simulink model "R7014E_QuadTankSim_LQG"  (R2025b)
settings: Solver=ode4  StartTime=0.0  StopTime=4000  FixedStep=0.01  RelTol=1e-3  EnableMultiTasking=on
values from neighbouring files (symbols this model uses):
  A1 = 28    [matlab_workspace.mat]
  a1 = 0.071    [matlab_workspace.mat]
  A2 = 32    [matlab_workspace.mat]
  a2 = 0.057    [matlab_workspace.mat]
  A3 = 28    [matlab_workspace.mat]
  a3 = 0.071    [matlab_workspace.mat]
  A4 = 32    [matlab_workspace.mat]
  a4 = 0.057    [matlab_workspace.mat]
  g = 981    [matlab_workspace.mat]
  gamma1 = 0.7    [matlab_workspace.mat]
  gamma1_M = 0.7    [matlab_workspace.mat]
  gamma2 = 0.6    [matlab_workspace.mat]
  gamma2_M = 0.6    [matlab_workspace.mat]
  h10_M = 12.3    [matlab_workspace.mat]
  h1_init = 12.3    [matlab_workspace.mat]
  h20_M = 12.8    [matlab_workspace.mat]
  h2_init = 12.8    [matlab_workspace.mat]
  h30_M = 1.6    [matlab_workspace.mat]
  h3_init = 1.6    [matlab_workspace.mat]
  h40_M = 1.4    [matlab_workspace.mat]
  h4_init = 1.4    [matlab_workspace.mat]
  k1 = 3.33    [matlab_workspace.mat]
  k1_M = 3.33    [matlab_workspace.mat]
  k2 = 3.35    [matlab_workspace.mat]
  k2_M = 3.35    [matlab_workspace.mat]
  L = [0.0253903063157  0.00669872251938  -0.00763717131985  17.1775356153; 0.0105780800885  0.0181633124943  21.4339038197  -0.0255525830892]    [matlab_workspace.mat]
  Lr = [4.62710191082  -2.40905188483; -3.22197937318  5.94561996641]    [matlab_workspace.mat]
  Q = gram(G_Pm,'o')    [Gramians_test.m]    (also in matlab_workspace.mat = [1e-08  0  0; 0  1e-08  0; 0  0  10])
  R = 0.1    [matlab_workspace.mat]
  Ts = 0.02    [matlab_workspace.mat]
  u_10_M = 3    [matlab_workspace.mat]
  u_20_M = 3    [matlab_workspace.mat]
undefined symbols (not defined in the file or in its folder): sigbuilder_block
Description:
  | Double tank process simulation model
  | V1.0
  | 
  | Author: Wolfgang Birk, LTU
settings Model: MinMaxOverflowLogging=ForceOff  Creator=wolfgang  LastModifiedBy=kaspe
settings SolverCC: AlgebraicLoopSolver=TrustRegion
settings DataIOCC: LimitDataPoints=on  SaveFormat=Array  SignalLoggingSaveFormat=ModelDataLogs  ReturnWorkspaceOutputs=off
settings OptimizationCC: ExpressionDepthLimit=2147483647.0  LifeSpan=inf
settings DebuggingCC: UnderspecifiedInitializationDetection=Classic  MergeDetectMultiDrivingBlocksExec=none  SolverPrmCheckMsg=warning  FcnCallInpInsideContextMsg=warning  UnconnectedInputMsg=warning  UnconnectedOutputMsg=warning  UnconnectedLineMsg=warning  StateNameClashWarn=warning  SFUnexpectedBacktrackingDiag=warning  SFNoUnconditionalDefaultTransitionDiag=warning  SFExecutionAtInitializationDiag=none  ArithmeticOperatorsInVariantConditions=warning
settings HardwareCC: ProdBitPerPointer=32.0  ProdBitPerSizeT=32.0  ProdBitPerPtrDiffT=32.0  ProdLargestAtomicFloat=None  ProdIntDivRoundTo=Undefined  ProdEndianess=Unspecified  ProdWordSize=32.0  ProdHWDeviceType=32-bit Generic
settings ModelReferenceCC: EnableRefExpFcnMdlSchedulingChecks=on  PropagateSignalLabelsOutOfModel=off
settings SFSimCC: SimUseLocalCustomCode=off  CustomCodeUndefinedFunction=UseInterfaceOnly
settings RTWCC: RTWUseLocalCustomCode=off  GPUComputeCapability=3.5
settings CodeAppCC: StateflowObjectComments=on
settings GRTTargetCC: TargetLangStandard=C89/C90 (ANSI)
settings ConfigComp: CovMetricSettings=dw  CovSaveCumulativeToWorkspaceVar=on  CovSaveSingleToWorkspaceVar=on  CovExternalEMLEnable=off

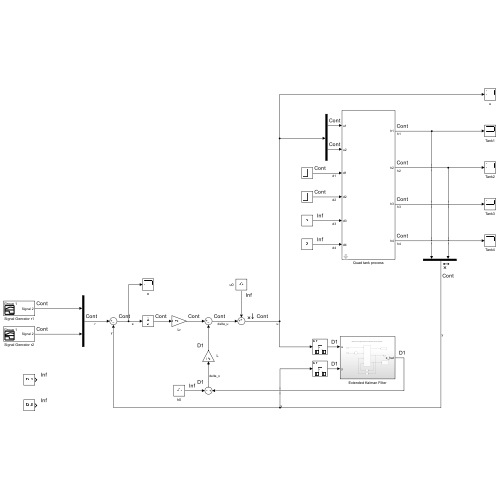
[thumbnail: Simulink's stored preview of the top-level diagram]
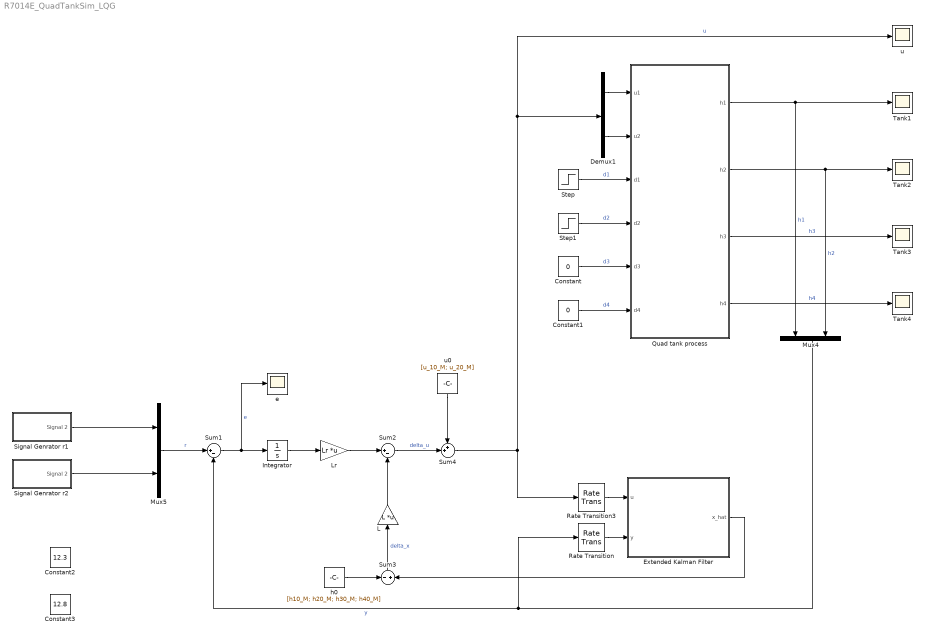
== system R7014E_QuadTankSim_LQG ==
  Constant : Constant  Value=0
  Constant1 : Constant  Value=0
  Constant2 : Constant  Value=12.3
  Constant3 : Constant  Value=12.8
  Demux1 : Demux  Outputs=2
  Extended Kalman Filter : Subsystem
      settings: PortSchema="{\"entries\":[{\"content\":{\"sides\":[{\"content\":{\"connectorIds\":[\"Out1\"]},\"type\":\"ConnectorPlacement.EquallySpacedRectSide\",\"uuid\":\"65fe89cb-b391-4b62-a3a2-a3476ef8bc40\"},{\"content\":{\"connectorIds\":[\"In1\",\"In2\"],\"side\":\"RIGHT\"},\"type\":\"ConnectorPlacement.EquallySpacedRectSide\",\"uuid\":\"bbc6305a-5625-4988-a68f-cd512a800022\"},{\"content\":{\"side\":\"TOP\"},\"type\":\"ConnectorPlacement.EquallySpacedRectSide\",\"uuid\":\"302c5684-92d4-4b6e-95b2-967c1f4e7e8f\"},{\"content\":{\"side\":\"BOTTOM\"},\"type\":\"ConnectorPlacement.EquallySpacedRectSide\",\"uuid\":\"8db0117f-7782-4a07-8d3a-766a48ad4692\"}]},\"type\":\"ConnectorPlacement.EquallySpacedConnector\",\"uuid\":\"a95b63f5-df7a-433e-a941-cc1845937f8d\"}],\"packageUris\":[\"http://schema.mathworks.com/mf0/Connector/R2020b\"],\"version\":\"1.0\"}"
  Integrator : Integrator
  L : Gain  Gain=L  Multiplication=Matrix(K*u)
  Lr : Gain  Gain=Lr  Multiplication=Matrix(K*u)
  Mux4 : Mux  Inputs=2
  Mux5 : Mux  Inputs=2
  Quad tank process : Subsystem  mask{hmax=20, A1=A1, ao1=a1, h10=h1_init, A2=A2, ao2=a2, h20=h2_init, A3=A3, ao3=a3, h30=h3_init, A4=A4, ao4=a4, h40=h4_init, k1=k1_M, k2=k2_M, gamma1=gamma1_M, gamma2=gamma2_M}
      mask prompts: hmax "Tank height (cm)"; A1 "Tank area (cm^2)"; ao1 "Opening area (cm^2)"; h10 "Initial level (cm)"; A2 "Tank area (cm^2)"; ao2 "Opening area (cm^2)"; h20 "Initial level (cm)"; A3 "Tank area (cm^2)"; ao3 "Opening area (cm^2)"; h30 "Initial level (cm)"; A4 "Tank area (cm^2)"; ao4 "Opening area (cm^2)"; h40 "Initial level (cm)"; k1 "Pump1 gain (cm^3/V/s)"; k2 "Pump2 gain (cm^3/V/s)"; gamma1 "Split valve gamma 1"; gamma2 "Split valve gamma 2"
      mask help: Double tank process parameters
      mask DialogControl Container3 Prompt: General parameters
      mask DialogControl ParameterGroupVar Prompt: Tank 1
      mask DialogControl ParameterGroupVar_copy_copy_copy Prompt: Tank 2
      mask DialogControl ParameterGroupVar_copy_copy Prompt: Tank 3
      mask DialogControl ParameterGroupVar_copy Prompt: Tank 4
      mask DialogControl Container4 Prompt: Pump parameters
  Rate Transition : RateTransition  InitialCondition=h1_init  OutPortSampleTime=Ts
  Rate Transition3 : RateTransition  InitialCondition=h2_init  OutPortSampleTime=Ts
  Signal Genrator r1 : Subsystem  Tag=STV Subsys  LoadFcn=sigbuilder_block('load');  StartFcn=sigbuilder_block('start');  StopFcn=sigbuilder_block('stop');  ClipboardFcn=sigbuilder_block('clipboard');  mask(Sigbuilder block){tuvar=[0:10]}
      mask help: Simulink:masks:SigbuilderBlock_MD
      mask init:
      | if ~strcmp(get_param(bdroot(gcbh),'SimulationStatus'),'stopped') tuvar = sigbuilder_block('maskInit'); end
      settings: CopyFcn=sigbuilder_block('copy');  DeleteFcn=sigbuilder_block('delete');  ModelCloseFcn=sigbuilder_block('modelClose');  PreSaveFcn=sigbuilder_block('preSave');  PauseFcn=sigbuilder_block('pause');  ContinueFcn=sigbuilder_block('continue');  NameChangeFcn=sigbuilder_block('namechange');  OpenFcn=sigbuilder_block('open',[289.5 231.75 954.75 575.25 ]);  CloseFcn=sigbuilder_block('close');
      mask Display: plot(0, 0, 100, 100,[2, 2, 32, 32, 2], [68, 8, 8, 68, 68],[32, 2], [38, 38], [32, 19, 2],[53, 60, 44], [32, 17, 17, 2],[16, 16, 31, 31]);txt = getActiveGroup(gcbh);text(2, 100, txt,'verticalAlignment', 'top');
  Signal Genrator r2 : Subsystem  Tag=STV Subsys  LoadFcn=sigbuilder_block('load');  StartFcn=sigbuilder_block('start');  StopFcn=sigbuilder_block('stop');  ClipboardFcn=sigbuilder_block('clipboard');  mask(Sigbuilder block){tuvar=[0:10]}
      mask help: Simulink:masks:SigbuilderBlock_MD
      mask init:
      | if ~strcmp(get_param(bdroot(gcbh),'SimulationStatus'),'stopped') tuvar = sigbuilder_block('maskInit'); end
      settings: CopyFcn=sigbuilder_block('copy');  DeleteFcn=sigbuilder_block('delete');  ModelCloseFcn=sigbuilder_block('modelClose');  PreSaveFcn=sigbuilder_block('preSave');  PauseFcn=sigbuilder_block('pause');  ContinueFcn=sigbuilder_block('continue');  NameChangeFcn=sigbuilder_block('namechange');  OpenFcn=sigbuilder_block('open',[289.5 231.75 954.75 575.25 ]);  CloseFcn=sigbuilder_block('close');
      mask Display: plot(0, 0, 100, 100,[2, 2, 32, 32, 2], [68, 8, 8, 68, 68],[32, 2], [38, 38], [32, 19, 2],[53, 60, 44], [32, 17, 17, 2],[16, 16, 31, 31]);txt = getActiveGroup(gcbh);text(2, 100, txt,'verticalAlignment', 'top');
  Step : Step  Time=1500  After=0.25  SampleTime=0
  Step1 : Step  Time=2700  After=0.25  SampleTime=0
  Sum1 : Sum  Inputs=|+-
  Sum2 : Sum  Inputs=|+-
  Sum3 : Sum  Inputs=-|+
  Sum4 : Sum  Inputs=++|
  Tank{1..4} (4 alike) : Scope
      Tank1 settings: TimeSpan=100  ActiveDisplayYMinimum=11.966385472015087  ActiveDisplayYMaximum=15.227429854493407
      Tank2 settings: TimeSpan=100  ActiveDisplayYMinimum=12.672164495001056  ActiveDisplayYMaximum=12.860911646500954  DataLoggingVariableName=ScopeData3
      Tank3 settings: TimeSpan=100  ActiveDisplayYMinimum=1.57505  ActiveDisplayYMaximum=1.66866
      Tank4 settings: TimeSpan=100  ActiveDisplayYMinimum=1.35987  ActiveDisplayYMaximum=1.45363  DataLoggingVariableName=ScopeData2
  e : Scope
      settings: TimeSpan=100  ActiveDisplayYMinimum=-0.93911904446836725  ActiveDisplayYMaximum=2.3265690426724981  DataLoggingVariableName=ScopeData8
  h0 : Constant  Value=[h10_M; h20_M; h30_M; h40_M]
  u : Scope
      settings: TimeSpan=100  ActiveDisplayYMinimum=-0.83563082318699256  ActiveDisplayYMaximum=10.21135105627962  DataLoggingVariableName=ScopeData4
  u0 : Constant  Value=[u_10_M; u_20_M]
  wires:
  Quad tank process/3(h3) -> Tank3/1  "h3"
  Quad tank process/1(h1) -> Tank1/1, Mux4/1  "h1"
  Step/1 -> Quad tank process/3(d1)  "d1"
  Step1/1 -> Quad tank process/4(d2)  "d2"
  Constant/1 -> Quad tank process/5(d3)  "d3"
  Constant1/1 -> Quad tank process/6(d4)  "d4"
  Quad tank process/2(h2) -> Tank2/1, Mux4/2  "h2"
  Quad tank process/4(h4) -> Tank4/1  "h4"
  Rate Transition/1 -> Extended Kalman Filter/1(y)
  Rate Transition3/1 -> Extended Kalman Filter/2(u)
  Extended Kalman Filter/1(x_hat) -> Sum3/2
  Mux4/1 -> Sum1/2, Rate Transition/1  "y"
  Demux1/1 -> Quad tank process/1(u1)
  Demux1/2 -> Quad tank process/2(u2)
  Mux5/1 -> Sum1/1  "r"
  L/1 -> Sum2/2
  Sum1/1 -> Integrator/1, e/1  "e"
  Sum3/1 -> L/1  "delta_x"
  h0/1 -> Sum3/1
  Sum2/1 -> Sum4/2  "delta_u"
  u0/1 -> Sum4/1
  Sum4/1 -> Rate Transition3/1, Demux1/1, u/1  "u"
  Signal Genrator r1/1(Signal 2) -> Mux5/1
  Signal Genrator r2/1(Signal 2) -> Mux5/2
  Lr/1 -> Sum2/1
  Integrator/1 -> Lr/1

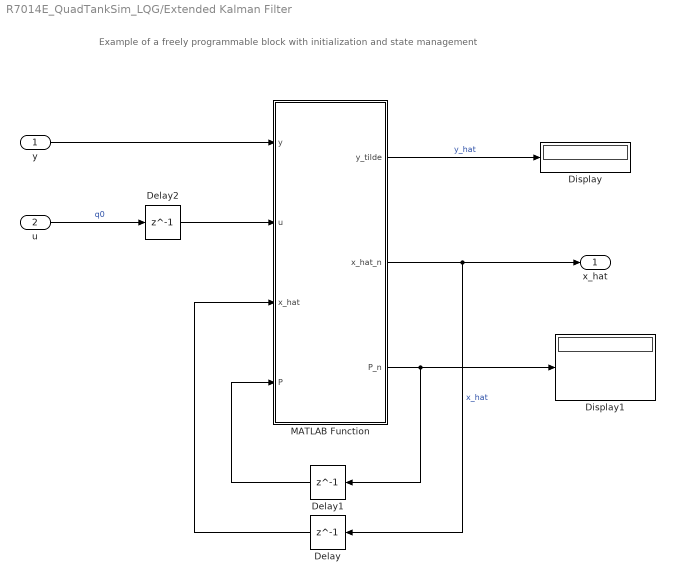
== system R7014E_QuadTankSim_LQG/Extended Kalman Filter ==
  note: Example of a freely programmable block with initialization and state management
  y : Inport
  u : Inport  Port=2
  Delay : Delay  DelayLength=1  InitialCondition=[h1_init, h2_init, h3_init, h4_init]
  Delay1 : Delay  DelayLength=1  InitialCondition=zeros(4)
  Delay2 : Delay  DelayLength=1  InitialCondition=0
  Display : Display
  Display1 : Display
  MATLAB Function : MATLAB Function  TreatAsAtomicUnit=on
  x_hat : Outport
  wires:
  Delay/1 -> MATLAB Function/3(x_hat)
  MATLAB Function/1(y_tilde) -> Display/1  "y_hat"
  MATLAB Function/3(P_n) -> Display1/1, Delay1/1
  Delay1/1 -> MATLAB Function/4(P)
  u/1 -> Delay2/1  "q0"
  MATLAB Function/2(x_hat_n) -> Delay/1, x_hat/1  "x_hat"
  Delay2/1 -> MATLAB Function/2(u)
  y/1 -> MATLAB Function/1(y)

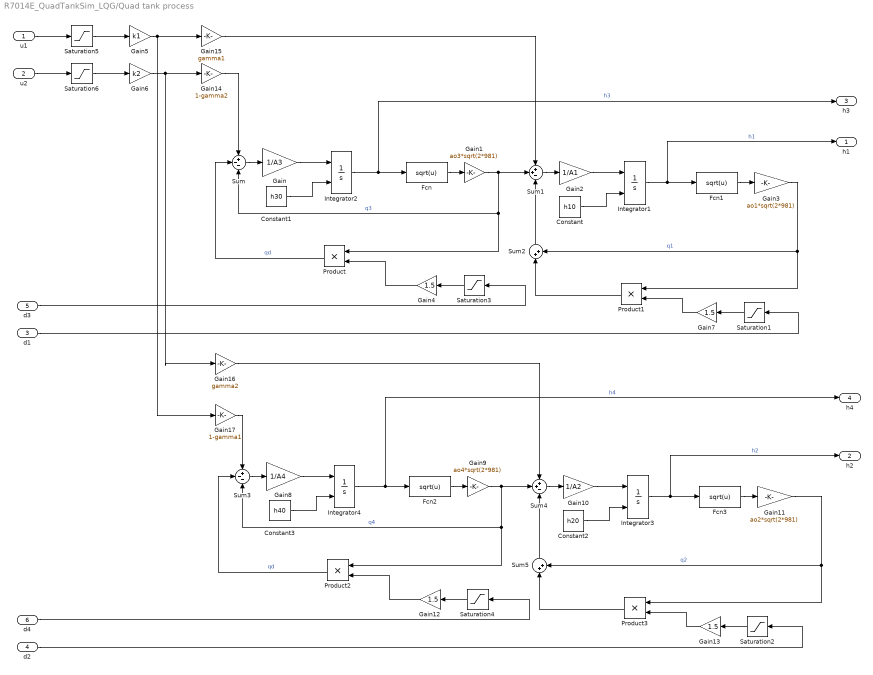
== system R7014E_QuadTankSim_LQG/Quad tank process ==
  u1 : Inport
  u2 : Inport  Port=2
  d1 : Inport  Port=3
  d2 : Inport  Port=4
  d3 : Inport  Port=5
  d4 : Inport  Port=6
  Constant : Constant  Value=h10
  Constant1 : Constant  Value=h30
  Constant2 : Constant  Value=h20
  Constant3 : Constant  Value=h40
  Fcn{,1..3} (4 alike) : Fcn  Expr=sqrt(u)
  Gain : Gain  Gain=1/A3
  Gain1 : Gain  Gain=ao3*sqrt(2*981)
  Gain10 : Gain  Gain=1/A2
  Gain11 : Gain  Gain=ao2*sqrt(2*981)
  Gain{4,7,12..13} (4 alike) : Gain  Gain=1.5
  Gain14 : Gain  Gain=1-gamma2
  Gain15 : Gain  Gain=gamma1
  Gain16 : Gain  Gain=gamma2
  Gain17 : Gain  Gain=1-gamma1
  Gain2 : Gain  Gain=1/A1
  Gain3 : Gain  Gain=ao1*sqrt(2*981)
  Gain5 : Gain  Gain=k1
  Gain6 : Gain  Gain=k2
  Gain8 : Gain  Gain=1/A4
  Gain9 : Gain  Gain=ao4*sqrt(2*981)
  Integrator{1..4} (4 alike) : Integrator  InitialConditionSource=external  LimitOutput=on  UpperSaturationLimit=hmax  LowerSaturationLimit=0
  Product{,1..3} (4 alike) : Product  RndMeth=Zero
  Saturation{1..4} (4 alike) : Saturate  UpperLimit=1  LowerLimit=0
  Saturation5 : Saturate  UpperLimit=10  LowerLimit=0
  Saturation6 : Saturate  UpperLimit=10  LowerLimit=0
  Sum : Sum  Inputs=+--
  Sum1 : Sum  Inputs=++-
  Sum2 : Sum  Inputs=|++
  Sum3 : Sum  Inputs=+--
  Sum4 : Sum  Inputs=++-
  Sum5 : Sum  Inputs=|++
  h1 : Outport  VectorParamsAs1DForOutWhenUnconnected=off
  h2 : Outport  Port=2  VectorParamsAs1DForOutWhenUnconnected=off
  h3 : Outport  Port=3  VectorParamsAs1DForOutWhenUnconnected=off
  h4 : Outport  Port=4  VectorParamsAs1DForOutWhenUnconnected=off
  wires:
  Sum/1 -> Gain/1
  Gain/1 -> Integrator2/1
  Fcn/1 -> Gain1/1
  Gain1/1 -> Product/1, Sum/3, Sum1/2  "q3"
  Sum1/1 -> Gain2/1
  Gain2/1 -> Integrator1/1
  Fcn1/1 -> Gain3/1
  Integrator2/1 -> h3/1, Fcn/1  "h3"
  Product/1 -> Sum/2  "qd"
  d3/1 -> Saturation3/1
  Integrator1/1 -> h1/1, Fcn1/1  "h1"
  Saturation3/1 -> Gain4/1
  Gain4/1 -> Product/2
  u1/1 -> Saturation5/1
  Constant/1 -> Integrator1/2
  Constant1/1 -> Integrator2/2
  u2/1 -> Saturation6/1
  Gain5/1 -> Gain17/1, Gain15/1
  Sum2/1 -> Sum1/3
  Gain3/1 -> Product1/1, Sum2/2  "q1"
  Gain7/1 -> Product1/2
  Saturation1/1 -> Gain7/1
  d1/1 -> Saturation1/1
  Product1/1 -> Sum2/1
  Product3/1 -> Sum5/1
  d2/1 -> Saturation2/1
  Saturation2/1 -> Gain13/1
  Gain13/1 -> Product3/2
  Gain11/1 -> Sum5/2, Product3/1  "q2"
  Sum5/1 -> Sum4/3
  Constant3/1 -> Integrator4/2
  Constant2/1 -> Integrator3/2
  Gain12/1 -> Product2/2
  Saturation4/1 -> Gain12/1
  Integrator3/1 -> Fcn3/1, h2/1  "h2"
  d4/1 -> Saturation4/1
  Product2/1 -> Sum3/2  "qd"
  Integrator4/1 -> h4/1, Fcn2/1  "h4"
  Fcn3/1 -> Gain11/1
  Gain10/1 -> Integrator3/1
  Sum4/1 -> Gain10/1
  Gain9/1 -> Sum4/2, Sum3/3, Product2/1  "q4"
  Fcn2/1 -> Gain9/1
  Gain8/1 -> Integrator4/1
  Sum3/1 -> Gain8/1
  Gain14/1 -> Sum/1
  Gain15/1 -> Sum1/1
  Gain6/1 -> Gain16/1, Gain14/1
  Gain16/1 -> Sum4/1
  Gain17/1 -> Sum3/1
  Saturation5/1 -> Gain5/1
  Saturation6/1 -> Gain6/1

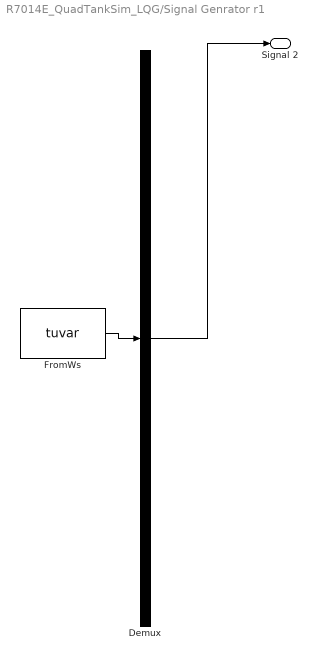
== system R7014E_QuadTankSim_LQG/Signal Genrator r1 ==
  Demux : Demux  Tag=STV Demux  Outputs=1
      settings: DisplayOption=none
  FromWs : FromWorkspace  Tag=STV FromWs  VariableName=tuvar
      SigBuilderData=|
      | common.afterFinalStr = 'Extrapolate'
      | common.sampleTime = 0
      | dataSet.timeRange = [0 2000]
      | dataSet.name = 'Group 1'
      | sbobj.Groups.Name = 'Group 1'
      | sbobj.Groups.Signals.Name = 'Signal 2'
      | sbobj.Groups.Signals.XData = [0 500 500 2000]
      | sbobj.Groups.Signals.YData = [12.3 12.3 14.3 14.3]
      | sbobj.Groups.TimeRange = [0 2000]
  Signal 2 : Outport  Tag=STV Outport
  wires:
  FromWs/1 -> Demux/1
  Demux/1 -> Signal 2/1

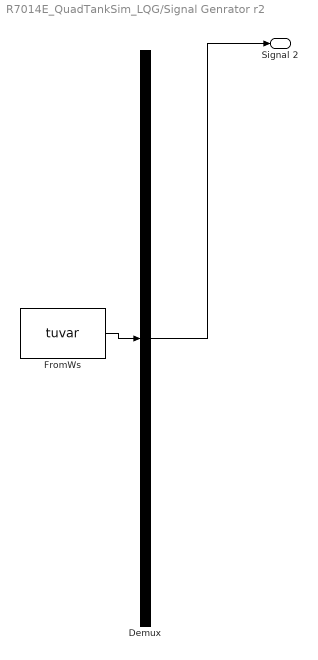
== system R7014E_QuadTankSim_LQG/Signal Genrator r2 ==
  Demux : Demux  Tag=STV Demux  Outputs=1
      settings: DisplayOption=none
  FromWs : FromWorkspace  Tag=STV FromWs  VariableName=tuvar
      SigBuilderData=|
      | common.afterFinalStr = 'Extrapolate'
      | common.sampleTime = 0
      | dataSet.timeRange = [0 2000]
      | dataSet.name = 'Group 1'
      | sbobj.Groups.Name = 'Group 1'
      | sbobj.Groups.Signals.Name = 'Signal 2'
      | sbobj.Groups.Signals.XData = [0 1000 1000 2000]
      | sbobj.Groups.Signals.YData = [12.8 12.8 14.8 14.8]
      | sbobj.Groups.TimeRange = [0 2000]
  Signal 2 : Outport  Tag=STV Outport
  wires:
  FromWs/1 -> Demux/1
  Demux/1 -> Signal 2/1

== matlab function R7014E_QuadTankSim_LQG/Extended Kalman Filter/MATLAB Function ==
  data: y input; u input; x_hat input; y_tilde output; x_hat_n output; P input; P_n output; Q parameter; R parameter; g parameter; Ts parameter; A1 parameter; A2 parameter; A3 parameter; A4 parameter; k1 parameter; k2 parameter; a1 parameter; a2 parameter; a3 parameter; a4 parameter; gamma1 parameter; gamma2 parameter
function [y_tilde, x_hat_n, P_n] = fcn(y, u, x_hat, P, Q, R, g, Ts, A1, A2, A3, A4, k1, k2, a1, a2, a3, a4, gamma1, gamma2)

h1_hat = x_hat(1);
h2_hat = x_hat(2);
h3_hat = x_hat(3);
h4_hat = x_hat(4);
Q = eye(4);
% Linearization


% Disturbances (Assumed zero for the filter's internal model unless estimated)
d1 = 0; d2 = 0; d3 = 0; d4 = 0;

% Safety margin to prevent division by zero if a tank empties
epsilon = 1e-6; 

%% Calculate State Jacobian Matrix (A)
A = zeros(4, 4);

A(1,1) = -((a1 + d1) / A1) * sqrt(g / (2 * max(h1_hat, epsilon)));
A(1,3) =  (a3 / A3) * sqrt(g / (2 * max(h3_hat, epsilon)));
A(2,2) = -((a2 + d2) / A2) * sqrt(g / (2 * max(h2_hat, epsilon)));
A(2,4) =  (a4 / A4) * sqrt(g / (2 * max(h4_hat, epsilon)));
A(3,3) = -((a3 + d3) / A3) * sqrt(g / (2 * max(h3_hat, epsilon)));
A(4,4) = -((a4 + d4) / A4) * sqrt(g / (2 * max(h4_hat, epsilon)));

%% Calculate Input Jacobian Matrix (B)
B = zeros(4, 2);

B(1,1) = (gamma1 * k1) / A1;
B(2,2) = (gamma2 * k2) / A2;
B(3,2) = ((1 - gamma2) * k2) / A3;
B(4,1) = ((1 - gamma1) * k1) / A4;

Ad = eye(size(A)) + Ts * A;

% Predict
sq1 = sqrt(2*g*max(h1_hat, epsilon));
sq2 = sqrt(2*g*max(h2_hat, epsilon));
sq3 = sqrt(2*g*max(h3_hat, epsilon));
sq4 = sqrt(2*g*max(h4_hat, epsilon));
x_hat_dot = [((-a1-d1)/A1*sq1 + a3/A3*sq3 + gamma1/A1*k1*u(1));
             ((-a2-d2)/A2*sq2 + a4/A4*sq4 + gamma2/A2*k2*u(2));
             ((-a3-d3)/A3*sq3 + (1-gamma2)/A3*k2*u(2));
             ((-a4-d4)/A4*sq4 + (1-gamma1)/A4*k1*u(1))];
x_hat_n = x_hat + x_hat_dot .* Ts;
P_n = Ad * P * Ad' + Q;

C = [1 0 0 0;
     0 1 0 0];

% Update
y_tilde = y - C * x_hat_n;
S = C * P_n * C' + R;
K = P_n * C' * inv(S);
x_hat_n = x_hat_n + K * y_tilde;
P_n = (eye(size(A)) - K * C) * P_n;   
y_tilde = y - C * x_hat_n;
